simulink model "ModeloSimulacion1"  (R2023a)
settings: Solver=VariableStepAuto  StartTime=0.0  StopTime=20.0  RelTol=1e-3
values from neighbouring files (symbols this model uses):
  d = 0.02    [Simulacion1.m]
  J = 2    [Simulacion1.m]
  Kb = 3    [Simulacion1.m]
  Kt = 2    [Simulacion1.m]
  L = 0.1    [Simulacion1.m]
  La = 3    [Simulacion1.m]
  M = 5    [Simulacion1.m]
  N = 2    [Simulacion1.m]
  R = 0.02    [Simulacion1.m]
  Ra = 6    [Simulacion1.m]
libraries: mobileRoboticsLib x1
settings Model: Creator=John_117  LastModifiedBy=John_117

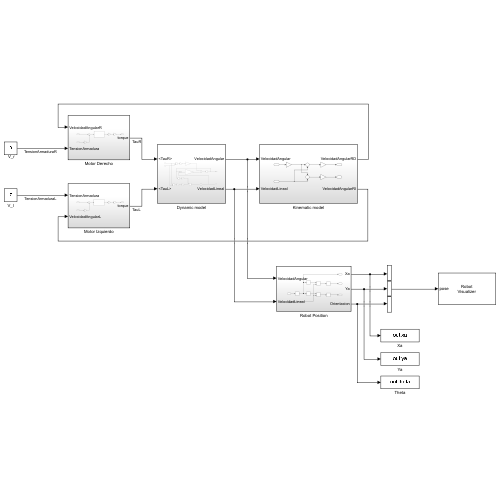
[thumbnail: Simulink's stored preview of the top-level diagram]
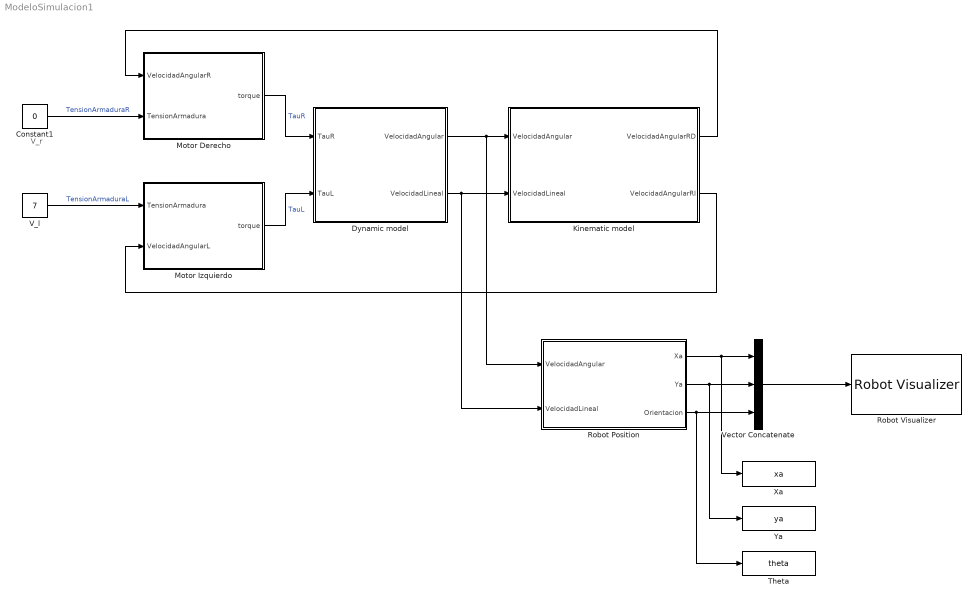
== system ModeloSimulacion1 ==
  note: V_r
  Constant1 : Constant  Value=0
  Dynamic model : Subsystem
  Kinematic model : Subsystem
  Motor Derecho : Subsystem
  Motor Izquierdo : Subsystem
  Robot Position : Subsystem
  Robot Visualizer : mobileRoboticsLib/Environments/Robot Visualizer  robotRadius=0  showTrajectory=on  hasWaypoints=off  hasLidar=off  sensorOffset=[ 0, 0 ]  scanAngles=[ -pi/4, 0, pi/4 ]  hasObjDetector=off  objDetectorOffset=[ 0, 0 ]  objDetectorAngle=0  objDetectorFOV=pi/4  objDetectorMaxRange=5  objectColors=[ 1, 0, 0; 0, 1, 0; 0, 0, 1 ]  objectMarkers=s
  Theta : ToWorkspace  VariableName=theta  SaveFormat=Timeseries  SampleTime=-1
      settings: Save2DSignal=2-D array (concatenate along first dimension)
  V_l : Constant  Value=7
  Vector Concatenate : Concatenate  NumInputs=3
  Xa : ToWorkspace  VariableName=xa  SaveFormat=Timeseries  SampleTime=-1
      settings: Save2DSignal=2-D array (concatenate along first dimension)
  Ya : ToWorkspace  VariableName=ya  SaveFormat=Timeseries  SampleTime=-1
      settings: Save2DSignal=2-D array (concatenate along first dimension)
  wires:
  Dynamic model/1(VelocidadAngular) -> Kinematic model/1(VelocidadAngular), Robot Position/1(VelocidadAngular)
  Dynamic model/2(VelocidadLineal) -> Kinematic model/2(VelocidadLineal), Robot Position/2(VelocidadLineal)
  Kinematic model/1(VelocidadAngularRD) -> Motor Derecho/1(VelocidadAngularR)
  Kinematic model/2(VelocidadAngularRI) -> Motor Izquierdo/2(VelocidadAngularL)
  Constant1/1 -> Motor Derecho/2(TensionArmadura)  "TensionArmaduraR"
  Motor Derecho/1(torque) -> Dynamic model/1(TauR)  "TauR"
  V_l/1 -> Motor Izquierdo/1(TensionArmadura)  "TensionArmaduraL"
  Motor Izquierdo/1(torque) -> Dynamic model/2(TauL)  "TauL"
  Robot Position/3(Orientacion) -> Theta/1, Vector Concatenate/3
  Robot Position/2(Ya) -> Ya/1, Vector Concatenate/2
  Robot Position/1(Xa) -> Vector Concatenate/1, Xa/1
  Vector Concatenate/1 -> Robot Visualizer/1

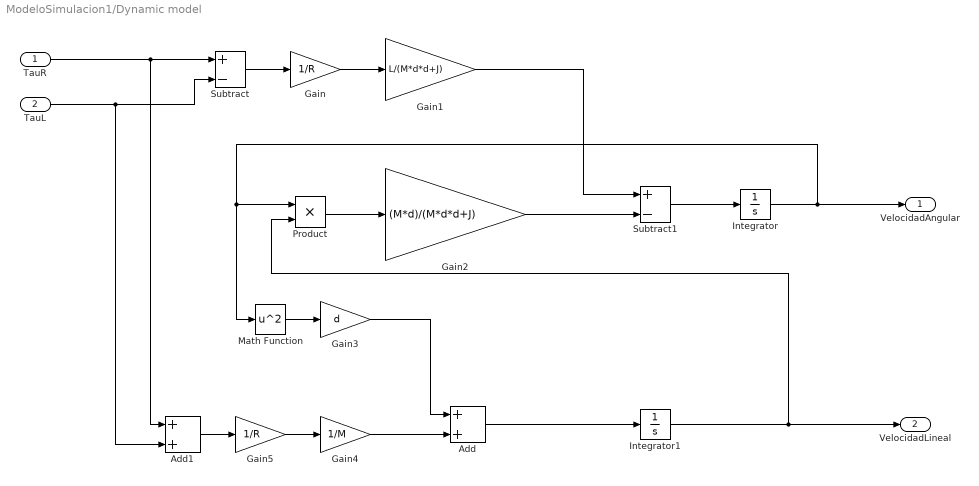
== system ModeloSimulacion1/Dynamic model ==
  TauR : Inport
  TauL : Inport  Port=2
  Add : Sum
  Add1 : Sum
  Gain : Gain  Gain=1/R
  Gain1 : Gain  Gain=L/(M*d*d+J)
  Gain2 : Gain  Gain=(M*d)/(M*d*d+J)
  Gain3 : Gain  Gain=d
  Gain4 : Gain  Gain=1/M
  Gain5 : Gain  Gain=1/R
  Integrator : Integrator
  Integrator1 : Integrator
  Math Function : Math  Operator=square
  Product : Product
  Subtract : Sum  Inputs=+-
  Subtract1 : Sum  Inputs=+-
  VelocidadAngular : Outport
  VelocidadLineal : Outport  Port=2
  wires:
  TauR/1 -> Add1/1, Subtract/1
  Gain4/1 -> Add/2
  Gain/1 -> Gain1/1
  Integrator/1 -> VelocidadAngular/1, Product/1, Math Function/1
  Integrator1/1 -> VelocidadLineal/1, Product/2
  Subtract1/1 -> Integrator/1
  Product/1 -> Gain2/1
  Gain1/1 -> Subtract1/1
  Gain5/1 -> Gain4/1
  Gain3/1 -> Add/1
  TauL/1 -> Add1/2, Subtract/2
  Math Function/1 -> Gain3/1
  Gain2/1 -> Subtract1/2
  Add1/1 -> Gain5/1
  Add/1 -> Integrator1/1
  Subtract/1 -> Gain/1

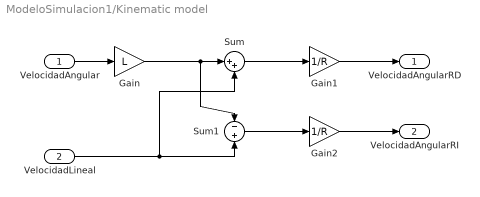
== system ModeloSimulacion1/Kinematic model ==
  VelocidadAngular : Inport
  VelocidadLineal : Inport  Port=2
  Gain : Gain  Gain=L
  Gain1 : Gain  Gain=1/R
  Gain2 : Gain  Gain=1/R
  Sum : Sum  Inputs=|++
  Sum1 : Sum  Inputs=-+
  VelocidadAngularRD : Outport
  VelocidadAngularRI : Outport  Port=2
  wires:
  Gain1/1 -> VelocidadAngularRD/1
  Sum1/1 -> Gain2/1
  Gain2/1 -> VelocidadAngularRI/1
  Gain/1 -> Sum/1, Sum1/1
  VelocidadLineal/1 -> Sum1/2, Sum/2
  VelocidadAngular/1 -> Gain/1
  Sum/1 -> Gain1/1

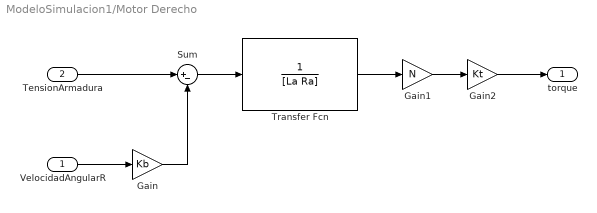
== system ModeloSimulacion1/Motor Derecho ==
  VelocidadAngularR : Inport
  TensionArmadura : Inport  Port=2
  Gain : Gain  Gain=Kb
  Gain1 : Gain  Gain=N
  Gain2 : Gain  Gain=Kt
  Sum : Sum  Inputs=|+-
  Transfer Fcn : TransferFcn  Denominator=[La Ra]
  torque : Outport
  wires:
  Sum/1 -> Transfer Fcn/1
  TensionArmadura/1 -> Sum/1
  Gain2/1 -> torque/1
  Gain/1 -> Sum/2
  Transfer Fcn/1 -> Gain1/1
  VelocidadAngularR/1 -> Gain/1
  Gain1/1 -> Gain2/1

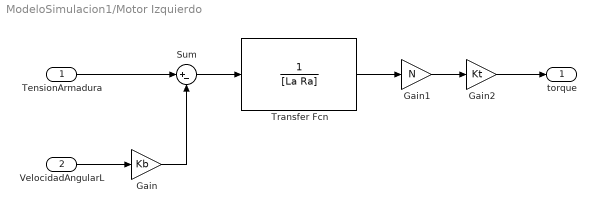
== system ModeloSimulacion1/Motor Izquierdo ==
  TensionArmadura : Inport
  VelocidadAngularL : Inport  Port=2
  Gain : Gain  Gain=Kb
  Gain1 : Gain  Gain=N
  Gain2 : Gain  Gain=Kt
  Sum : Sum  Inputs=|+-
  Transfer Fcn : TransferFcn  Denominator=[La Ra]
  torque : Outport
  wires:
  Sum/1 -> Transfer Fcn/1
  TensionArmadura/1 -> Sum/1
  Gain2/1 -> torque/1
  Gain/1 -> Sum/2
  Transfer Fcn/1 -> Gain1/1
  VelocidadAngularL/1 -> Gain/1
  Gain1/1 -> Gain2/1

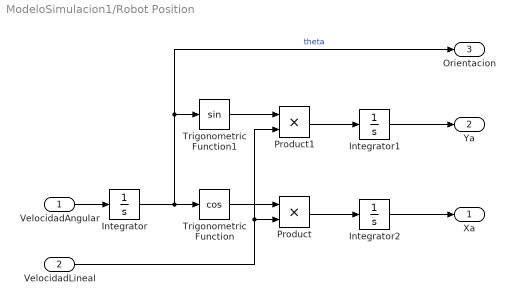
== system ModeloSimulacion1/Robot Position ==
  VelocidadAngular : Inport
  VelocidadLineal : Inport  Port=2
  Integrator : Integrator
  Integrator1 : Integrator
  Integrator2 : Integrator
  Product : Product
  Product1 : Product
  Trigonometric Function : Trigonometry  Operator=cos
  Trigonometric Function1 : Trigonometry
  Xa : Outport
  Ya : Outport  Port=2
  Orientacion : Outport  Port=3
  wires:
  Integrator1/1 -> Ya/1
  VelocidadAngular/1 -> Integrator/1
  Integrator2/1 -> Xa/1
  Integrator/1 -> Orientacion/1, Trigonometric Function1/1, Trigonometric Function/1  "theta"
  Product1/1 -> Integrator1/1
  Trigonometric Function/1 -> Product/1
  VelocidadLineal/1 -> Product1/2, Product/2
  Product/1 -> Integrator2/1
  Trigonometric Function1/1 -> Product1/1
